simulink library "Disabled_lib"  (R2023b)
settings: Solver=VariableStepAuto  StartTime=0.0  StopTime=10.0  RelTol=1e-3
undefined symbols (not defined in the file): Spline_Num_Poses_default, Spline_Ref_Poses_default
settings Model: Creator=FIRSTMentor  LastModifiedBy=ander

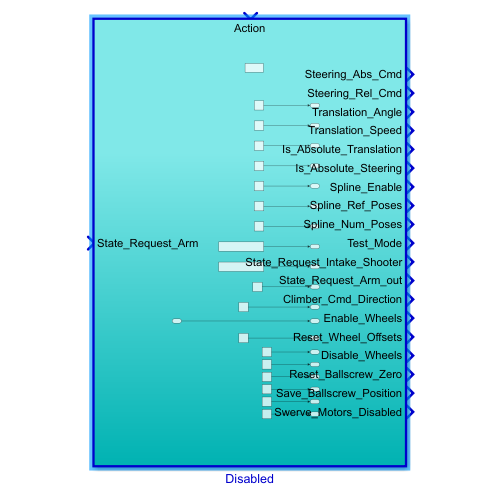
[thumbnail: Simulink's stored preview of the top-level diagram]
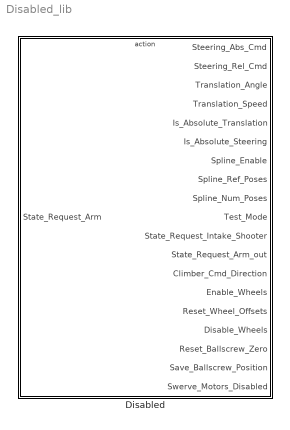
== system Disabled_lib ==
  Disabled : Subsystem  TreatAsAtomicUnit=on

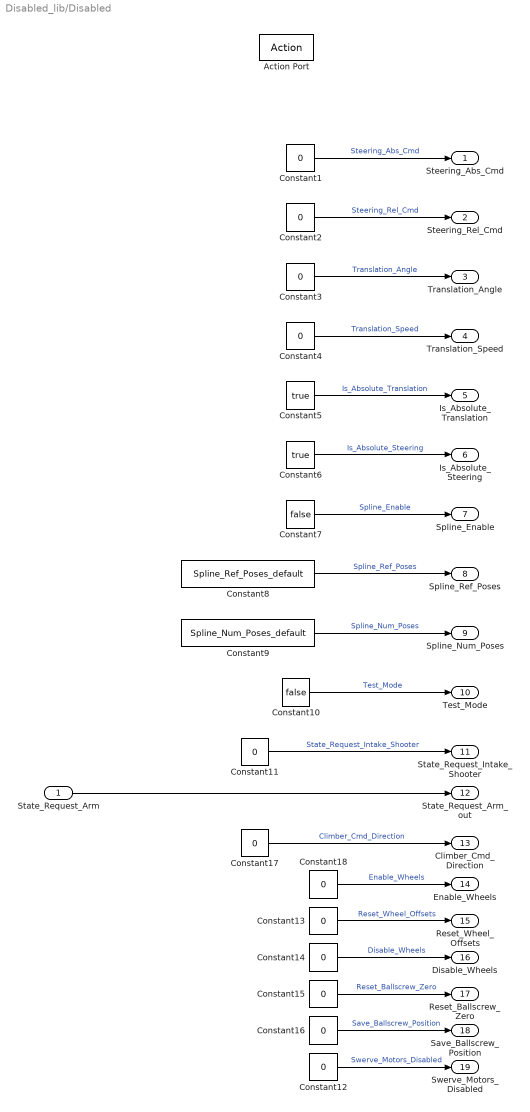
== system Disabled_lib/Disabled ==
  State_Request_Arm : Inport
  Action Port : ActionPort
  Constant{1..4,11,13..18} (11 alike) : Constant  Value=0
  Constant10 : Constant  Value=false  OutDataTypeStr=boolean
  Constant12 : Constant  Value=0  OutDataTypeStr=boolean
  Constant5 : Constant  Value=true
  Constant6 : Constant  Value=true
  Constant7 : Constant  Value=false  OutDataTypeStr=boolean
  Constant8 : Constant  Value=Spline_Ref_Poses_default
  Constant9 : Constant  Value=Spline_Num_Poses_default  OutDataTypeStr=double
  Steering_Abs_Cmd : Outport
  Steering_Rel_Cmd : Outport  Port=2
  Translation_Angle : Outport  Port=3
  Translation_Speed : Outport  Port=4
  Is_Absolute_Translation : Outport  Port=5
  Is_Absolute_Steering : Outport  Port=6
  Spline_Enable : Outport  Port=7
  Spline_Ref_Poses : Outport  Port=8
  Spline_Num_Poses : Outport  Port=9
  Test_Mode : Outport  Port=10
  State_Request_Intake_Shooter : Outport  Port=11
  State_Request_Arm_out : Outport  Port=12
  Climber_Cmd_Direction : Outport  Port=13
  Enable_Wheels : Outport  Port=14
  Reset_Wheel_Offsets : Outport  Port=15
  Disable_Wheels : Outport  Port=16
  Reset_Ballscrew_Zero : Outport  Port=17
  Save_Ballscrew_Position : Outport  Port=18
  Swerve_Motors_Disabled : Outport  Port=19
  wires:
  Constant1/1 -> Steering_Abs_Cmd/1  "Steering_Abs_Cmd"
  Constant2/1 -> Steering_Rel_Cmd/1  "Steering_Rel_Cmd"
  Constant3/1 -> Translation_Angle/1  "Translation_Angle"
  Constant4/1 -> Translation_Speed/1  "Translation_Speed"
  Constant5/1 -> Is_Absolute_Translation/1  "Is_Absolute_Translation"
  Constant6/1 -> Is_Absolute_Steering/1  "Is_Absolute_Steering"
  Constant7/1 -> Spline_Enable/1  "Spline_Enable"
  Constant8/1 -> Spline_Ref_Poses/1  "Spline_Ref_Poses"
  Constant9/1 -> Spline_Num_Poses/1  "Spline_Num_Poses"
  Constant10/1 -> Test_Mode/1  "Test_Mode"
  Constant11/1 -> State_Request_Intake_Shooter/1  "State_Request_Intake_Shooter"
  Constant17/1 -> Climber_Cmd_Direction/1  "Climber_Cmd_Direction"
  State_Request_Arm/1 -> State_Request_Arm_out/1
  Constant16/1 -> Save_Ballscrew_Position/1  "Save_Ballscrew_Position"
  Constant14/1 -> Disable_Wheels/1  "Disable_Wheels"
  Constant15/1 -> Reset_Ballscrew_Zero/1  "Reset_Ballscrew_Zero"
  Constant13/1 -> Reset_Wheel_Offsets/1  "Reset_Wheel_Offsets"
  Constant12/1 -> Swerve_Motors_Disabled/1  "Swerve_Motors_Disabled"
  Constant18/1 -> Enable_Wheels/1  "Enable_Wheels"
